simulink model "UpSamplingDemo"  (Simulink 6.3)
settings: Solver=FixedStepDiscrete  StartTime=0.0  StopTime=70  FixedStep=1  RelTol=1e-3
InitFcn:
  | %% DSPBuilder Start
  | alt_dspbuilder_update_model(bdroot)
  | %% DSPBuilder End
libraries: allblocks_alteradspbuilder2 x6
settings Model: LastModifiedBy=delphick
settings OptimizationCC: BlockReduction=off  BooleanDataType=off  InlineInvariantSignals=on
settings DebuggingCC: SolverPrmCheckMsg=none
settings HardwareCC: TargetUnknown=on

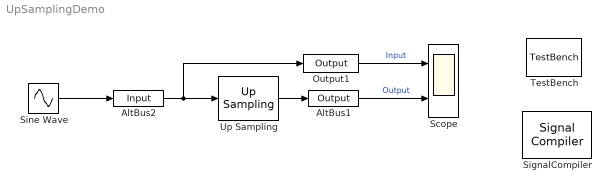
== system UpSamplingDemo ==
  AltBus1 : allblocks_alteradspbuilder2/Output  iofile=C:\workspace_clean\Documentation\DesignExamples\Tutorials\UnitBlocks\Storage\UpSampling\tb_UpSamplingDemo\UpSamplingDemo_AltBus1.capture  BusType=Signed Integer  bwl=5  bwr=4  PORTTYPE=Output
  AltBus2 : allblocks_alteradspbuilder2/Input  iofile=C:\workspace_clean\Documentation\DesignExamples\Tutorials\UnitBlocks\Storage\UpSampling\tb_UpSamplingDemo\UpSamplingDemo_AltBus2.salt  BusType=Signed Integer  bwl=5  bwr=4  SpecifyClock=off  PORTTYPE=Input
  Output1 : allblocks_alteradspbuilder2/Output  iofile=C:\workspace_clean\Documentation\DesignExamples\Tutorials\UnitBlocks\Storage\UpSampling\tb_UpSamplingDemo\UpSamplingDemo_Output1.capture  BusType=Signed Integer  bwl=5  bwr=0  PORTTYPE=Output
  Scope : Scope  NumInputPorts=2
      settings: YMin=-10~-10  YMax=10~10
  SignalCompiler : allblocks_alteradspbuilder2/Signal Compiler  DeviceFamily=Stratix IV  DeviceName=AUTO  EnableSignalTap=off  SignalTapDepth=128  UseBoardBlock=off  StpUseDefaultClock=on  StpClock=clock
  Sine Wave : Sin  Amplitude=8  Frequency=0.1  SampleTime=1
  TestBench : allblocks_alteradspbuilder2/TestBench  enable=on  advancedMode=on  modelSimGui=off  simdatafile=C:\workspace_clean\Documentation\DesignExamples\Tutorials\UnitBlocks\Storage\UpSampling\tb_UpSamplingDemo\UpSamplingDemo.simdata.tcl
  Up Sampling : allblocks_alteradspbuilder2/Up Sampling  rate=4
  wires:
  AltBus1/1 -> Scope/2  "Output"
  Up Sampling/1 -> AltBus1/1
  Sine Wave/1 -> AltBus2/1
  AltBus2/1 -> Up Sampling/1, Output1/1
  Output1/1 -> Scope/1  "Input"
